simulink model "draft7"  (R2023a)
settings: Solver=VariableStepAuto  StartTime=0.0  StopTime=10  FixedStep=0.0001  MaxStep=0.1  RelTol=1e-3  AbsTol=1e-3  EnableMultiTasking=on
model workspace (MAT data in the model file):
  C_Gimbal = 0.1
  C_IAP = 0.01
  IAP_Pa = 0
  K_Gimbal = 0
  K_IAP = 10
  LeftAbdominalMuscleForce = 0
  LeftBackMuscleForce = 0
  LeftTransverse1MuscleForce = 0
  LeftTransverse2MuscleForce = 0
  Moment_AR = 0
  Moment_FE = 0
  Moment_LB = 0
  RightAbdominalMuscleForce = 0
  RightBackMuscleForce = 0
  RightTransverse1MuscleForce = 0
  RightTransverse2MuscleForce = 0
  a = 1
  b = 1
undefined symbols (not defined in the file): X, Y, Z
libraries: sm_lib x279, nesl_utility x233, simulink_extras x33, checkpacklib x3, simulink x1
(part 2 of 7)

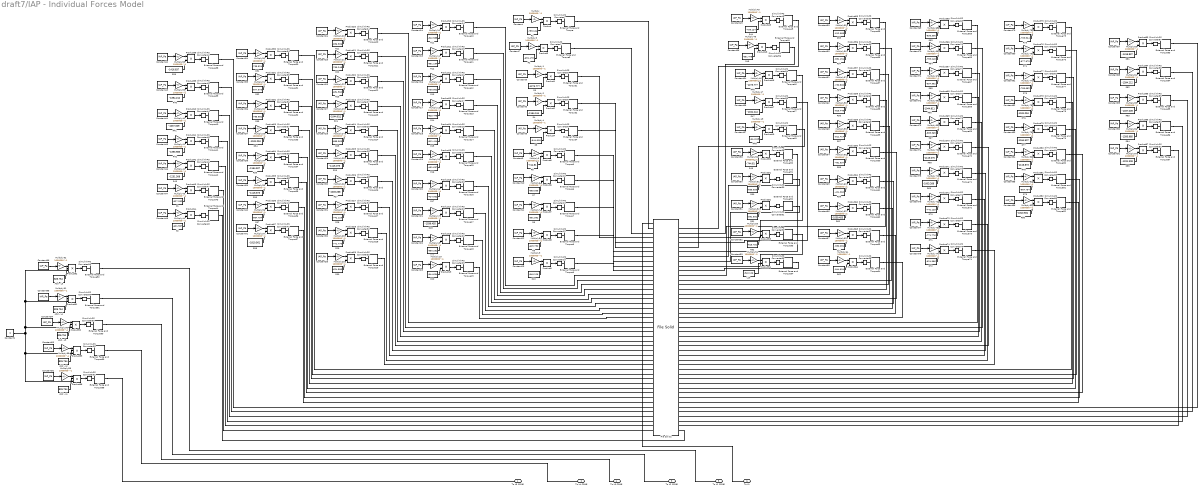
== system draft7/IAP - Individual Forces Model ==
  Abd - L{1..5} (5 alike) : Constant  Value=826.754
  C1 : Constant  Value=-527.332
  C2 : Constant  Value=-621.907
  Constant{,5..96} (93 alike) : Constant  Value=IAP_Pa
  Constant1 : Constant
  External Force and Torque{,1..92} (93 alike) : sm_lib/Forces and Torques/External Force and Torque  ForceResolutionFrame=AttachedFrame  EnableForceX=off  EnableForceY=off  EnableForceZ=on  EnableForce=off  TorqueResolutionFrame=AttachedFrame  EnableTorqueX=off  EnableTorqueY=off  EnableTorqueZ=off  EnableTorque=off
  File Solid2 : sm_lib/Body Elements/File Solid  ExtGeomFileName=C:\Users\siril\OneDrive\Desktop\TIM-Control\Matlab\Simscape models\CAD - with COM\SymmetricModel\draft7\Abd-diamond-flat-solid.step  UnitType=FromFile  ExtGeomFileUnits=m  StepReaderType=HEX  ExportConvexHullGeometry=off  InertiaType=CalculateFromGeometry  Mass=1  MassUnits=kg  CenterOfMass=[0 0 0]  CenterOfMassUnits=m  MomentsOfInertia=[1 1 1]  MomentsOfInertiaUnits=kg*m^2  ProductsOfInertia=[0 0 0]  ProductsOfInertiaUnits=kg*m^2  BasedOnType=Density  Density=0.182  DensityUnits=g/cm^3  DoExposeReferenceFrame=on  SerializedFrames=<Frames><Frame><Id>Frame1</Id><Value><Name>To L1</Name><Origin><Source>GeometricFeature</Source><FeatureName>planar surface 723</FeatureName></Origin><PrimaryAxis><DefinedDirection>-Z</DefinedDirection><Source>GeometricFeature</Source><SourceDirection>+Z</SourceDirection><FeatureName>planar surface 723</FeatureName></PrimaryAxis><SecondaryAxis><DefinedDirection>+X</DefinedDirection><Source>ReferenceFrame</Source><SourceDirection>+X</SourceDirection><FeatureName></FeatureName></SecondaryAxis></Value></Frame><Frame><Id>Frame2</Id><Value><Name>L1</Name><Origin><Source>GeometricFeature</Source><FeatureName>planar surface 1442</FeatureName></Origin><PrimaryAxis><DefinedDirection>+Z</DefinedDirection><Source>GeometricFeature</Source><SourceDirection>+Z</SourceDirection><FeatureName>planar surface 1442</FeatureName></PrimaryAxis><SecondaryAxis><DefinedDirection>+X</DefinedDirection><Source>ReferenceFrame</Source><SourceDirection>+X</SourceDirection><FeatureName></FeatureName></SecondaryAxis></Value></Frame><Frame><Id>Frame3</Id><Value><Name>R1</Name><Origin><Source>GeometricFeature</Source><FeatureName>planar surface 707</FeatureName></Origin><PrimaryAxis><DefinedDirection>-Z</DefinedDirection><Source>GeometricFeature</Source><SourceDirection>+Z</SourceDirection><FeatureName>planar surface 707</FeatureName></PrimaryAxis><SecondaryAxis><DefinedDirection>+X</DefinedDirection><Source>ReferenceFrame</Source><SourceDirection>+X</SourceDirection><FeatureName></FeatureName></SecondaryAxis></Value></Frame><Frame><Id>Frame4</Id><Value><Name>L2</Name><Origin><Source>GeometricFeature</Source><FeatureName>planar surface 1450</FeatureName></Origin><PrimaryAxis><DefinedDirection>+Z</DefinedDirection><Source>GeometricFeature</Source><SourceDirection>+Z</SourceDirection><FeatureName>planar surface 1450</FeatureName></PrimaryAxis><SecondaryAxis><DefinedDirection>+X</DefinedDirection><Source>ReferenceFrame</Source><SourceDirection>+X</SourceDirection><FeatureName></FeatureName></SecondaryAxis></Value></Frame><Frame><Id>Frame5</Id><Value><Name>R2</Name><Origin><Source>GeometricFeature</Source><FeatureName>planar surface 715</FeatureName></Origin><PrimaryAxis><DefinedDirection>-Z</DefinedDirection><Source>GeometricFeature</Source><SourceDirection>+Z</SourceDirection><FeatureName>planar surface 715</FeatureName></PrimaryAxis><SecondaryAxis><DefinedDirection>+X</DefinedDirection><Source>ReferenceFrame</Source><SourceDirection>+X</SourceDirection><FeatureName></FeatureName></SecondaryAxis></Value></Frame><Frame><Id>Frame6</Id><Value><Name>L3</Name><Origin><Source>GeometricFeature</Source><FeatureName>planar surface 1412</FeatureName></Origin><PrimaryAxis><DefinedDirection>+Z</DefinedDirection><Source>GeometricFeature</Source><SourceDirection>+Z</SourceDirection><FeatureName>planar surface 1412</FeatureName></PrimaryAxis><SecondaryAxis><DefinedDirection>+X</DefinedDirection><Source>ReferenceFrame</Source><SourceDirection>+X</SourceDirection><FeatureName></FeatureName></SecondaryAxis></Value></Frame><Frame><Id>Frame7</Id><Value><Name>R3</Name><Origin><Source>GeometricFeature</Source><FeatureName>planar surface 677</FeatureName></Origin><PrimaryAxis><DefinedDirection>-Z</DefinedDirection><Source>GeometricFeature</Source><SourceDirection>+Z</SourceDirection><FeatureName>planar surface 677</FeatureName></PrimaryAxis><SecondaryAxis><DefinedDirection>+X</DefinedDirection><Source>ReferenceFrame</Source><SourceDirection>+X</SourceDirection><FeatureName></FeatureName></SecondaryAxis></Value></Frame><Frame><Id>Frame8</Id><Value><Name>L4</Name><Origin><Source>GeometricFeature</Source><FeatureName>planar surface 1159</FeatureName></Origin><PrimaryAxis><DefinedDirection>+Z</DefinedDirection><Source>GeometricFeature</Source><SourceDirection>+Z</SourceDirection><FeatureName>planar surface 1159</FeatureName></PrimaryAxis><SecondaryAxis><DefinedDirection>+X</DefinedDirection><Source>ReferenceFrame</Source><SourceDirection>+X</SourceDirection><FeatureName></FeatureName></SecondaryAxis></Value></Frame><Frame><Id>Frame9</Id><Value><Name>R4</Name><Origin><Source>GeometricFeature</Source><FeatureName>planar surface 431</FeatureName></Origin><PrimaryAxis><DefinedDirection>-Z</DefinedDirection><Source>GeometricFeature</Source><SourceDirection>+Z</SourceDirection><FeatureName>planar surface 431</FeatureName></PrimaryAxis><SecondaryAxis><DefinedDirection>+X</DefinedDirection><Source>ReferenceFrame</Source><SourceDirection>+X</SourceDirection><FeatureName></FeatureName></SecondaryAxis></Value></Frame><Frame><Id>Frame10</Id><Value><Name>L5</Name><Origin><Source>GeometricFeature</Source><FeatureName>planar surface 1433</FeatureName></Origin><PrimaryAxis><DefinedDirection>+Z</DefinedDirection><Source>GeometricFeature</Source><SourceDirection>+Z</SourceDirection><FeatureName>planar surface 1433</FeatureName></PrimaryAxis><SecondaryAxis><DefinedDirection>+X</DefinedDirection><Source>ReferenceFrame</Source><SourceDirection>+X</SourceDirection><FeatureName></FeatureName></SecondaryAxis></Value></Frame><Frame><Id>Frame11</Id><Value><Name>R5</Name><Origin><Source>GeometricFeature</Source><FeatureName>planar surface 698</FeatureName></Origin><PrimaryAxis><DefinedDirection>-Z</DefinedDirection><Source>GeometricFeature</Source><SourceDirection>+Z</SourceDirection><FeatureName>planar surface 698</FeatureName></PrimaryAxis><SecondaryAxis><DefinedDirection>+X</DefinedDirection><Source>ReferenceFrame</Source><SourceDirection>+X</SourceDirection><FeatureName></FeatureName></SecondaryAxis></Value></Frame><Frame><Id>Frame12</Id><Value><Name>L6</Name><Origin><Source>GeometricFeature</Source><FeatureName>planar surface 1135</FeatureName></Origin><PrimaryAxis><DefinedDirection>+Z</DefinedDirection><Source>GeometricFeature</Source><SourceDirection>+Z</SourceDirection><FeatureName>planar surface 1135</FeatureName></PrimaryAxis><SecondaryAxis><DefinedDirection>+X</DefinedDirection><Source>ReferenceFrame</Source><SourceDirection>+X</SourceDirection><FeatureName></FeatureName></SecondaryAxis></Value></Frame><Frame><Id>Frame13</Id><Value><Name>R6</Name><Origin><Source>GeometricFeature</Source><FeatureName>planar surface 407</FeatureName></Origin><PrimaryAxis><DefinedDirection>-Z</DefinedDirection><Source>GeometricFeature</Source><SourceDirection>+Z</SourceDirection><FeatureName>planar surface 407</FeatureName></PrimaryAxis><SecondaryAxis><DefinedDirection>+X</DefinedDirection><Source>ReferenceFrame</Source><SourceDirection>+X</SourceDirection><FeatureName></FeatureName></SecondaryAxis></Value></Frame><Frame><Id>Frame14</Id><Value><Name>L7</Name><Origin><Source>GeometricFeature</Source><FeatureName>planar surface 1217</FeatureName></Origin><PrimaryAxis><DefinedDirection>+Z</DefinedDirection><Source>GeometricFeature</Source><SourceDirection>+Z</SourceDirection><FeatureName>planar surface 1217</FeatureName></PrimaryAxis><SecondaryAxis><DefinedDirection>+X</DefinedDirection><Source>ReferenceFrame</Source><SourceDirection>+X</SourceDirection><FeatureName></FeatureName></SecondaryAxis></Value></Frame><Frame><Id>Frame15</Id><Value><Name>R7</Name><Origin><Source>GeometricFeature</Source><FeatureName>planar surface 482</FeatureName></Origin><PrimaryAxis><DefinedDirection>-Z</DefinedDirection><Source>GeometricFeature</Source><SourceDirection>+Z</SourceDirection><FeatureName>planar surface 482</FeatureName></PrimaryAxis><SecondaryAxis><DefinedDirection>+X</DefinedDirection><Source>ReferenceFrame</Source><SourceDirection>+X</SourceDirection><FeatureName></FeatureName></SecondaryAxis></Value></Frame><Frame><Id>Frame16</Id><Value><Name>L8</Name><Origin><Source>GeometricFeature</Source><FeatureName>planar surface 1125</FeatureName></Origin><PrimaryAxis><DefinedDirection>+Z</DefinedDirection><Source>GeometricFeature</Source><SourceDirection>+Z</SourceDirection><FeatureName>planar surface 1125</FeatureName></PrimaryAxis><SecondaryAxis><DefinedDirection>+X</DefinedDirection><Source>ReferenceFrame</Source><SourceDirection>+X</SourceDirection><FeatureName></FeatureName></SecondaryAxis></Value></Frame><Frame><Id>Frame17</Id><Value><Name>R8</Name><Origin><Source>GeometricFeature</Source><FeatureName>planar surface 397</FeatureName></Origin><PrimaryAxis><DefinedDirection>-Z</DefinedDirection><Source>GeometricFeature</Source><SourceDirection>+Z</SourceDirection><FeatureName>planar surface 397</FeatureName></PrimaryAxis><SecondaryAxis><DefinedDirection>+X</DefinedDirection><Source>ReferenceFrame</Source><SourceDirection>+X</SourceDirection><FeatureName></FeatureName></SecondaryAxis></Value></Frame><Frame><Id>Frame18</Id><Value><Name>L9</Name><Origin><Source>GeometricFeature</Source><FeatureName>planar surface 1123</FeatureName></Origin><PrimaryAxis><DefinedDirection>+Z</DefinedDirection><Source>GeometricFeature</Source><SourceDirection>+Z</SourceDirection><FeatureName>planar surface 1123</FeatureName></PrimaryAxis><SecondaryAxis><DefinedDirection>+X</DefinedDirection><Source>ReferenceFrame</Source><SourceDirection>+X</SourceDirection><FeatureName></FeatureName></SecondaryAxis></Value></Frame><Frame><Id>Frame19</Id><Value><Name>R9</Name><Origin><Source>GeometricFeature</Source><FeatureName>planar surface 395</FeatureName></Origin><PrimaryAxis><DefinedDirection>-Z</DefinedDirection><Source>GeometricFeature</Source><SourceDirection>+Z</SourceDirection><FeatureName>planar surface 395</FeatureName></PrimaryAxis><SecondaryAxis><DefinedDirection>+X</DefinedDirection><Source>ReferenceFrame</Source><SourceDirection>+X</SourceDirection><FeatureName></FeatureName></SecondaryAxis></Value></Frame><Frame><Id>Frame20</Id><Value><Name>L10</Name><Origin><Source>GeometricFeature</Source><FeatureName>planar surface 1120</FeatureName></Origin><PrimaryAxis><DefinedDirection>+Z</DefinedDirection><Source>GeometricFeature</Source><SourceDirection>+Z</SourceDirection><FeatureName>planar surface 1120</FeatureName></PrimaryAxis><SecondaryAxis><DefinedDirection>+X</DefinedDirection><Source>ReferenceFrame</Source><SourceDirection>+X</SourceDirection><FeatureName></FeatureName></SecondaryAxis></Value></Frame><Frame><Id>Frame21</Id><Value><Name>R10</Name><Origin><Source>GeometricFeature</Source><FeatureName>planar surface 392</FeatureName></Origin><PrimaryAxis><DefinedDirection>-Z</DefinedDirection><Source>GeometricFeature</Source><SourceDirection>+Z</SourceDirection><FeatureName>planar surface 392</FeatureName></PrimaryAxis><SecondaryAxis><DefinedDirection>+X</DefinedDirection><Source>ReferenceFrame</Source><SourceDirection>+X</SourceDirection><FeatureName></FeatureName></SecondaryAxis></Value></Frame><Frame><Id>Frame22</Id><Value><Name>L11</Name><Origin><Source>GeometricFeature</Source><FeatureName>planar surface 1182</FeatureName></Origin><PrimaryAxis><DefinedDirection>+Z</DefinedDirection><Source>GeometricFeature</Source><SourceDirection>+Z</SourceDirection><FeatureName>planar surface 1182</FeatureName></PrimaryAxis><SecondaryAxis><DefinedDirection>+X</DefinedDirection><Source>ReferenceFrame</Source><SourceDirection>+X</SourceDirection><FeatureName></FeatureName></SecondaryAxis></Value></Frame><Frame><Id>Frame23</Id><Value><Name>R11</Name><Origin><Source>GeometricFeature</Source><FeatureName>planar surface 452</FeatureName></Origin><PrimaryAxis><DefinedDirection>-Z</DefinedDirection><Source>GeometricFeature</Source><SourceDirection>+Z</SourceDirection><FeatureName>planar surface 452</FeatureName></PrimaryAxis><SecondaryAxis><DefinedDirection>+X</DefinedDirection><Source>ReferenceFrame</Source><SourceDirection>+X</SourceDirection><FeatureName></FeatureName></SecondaryAxis></Value></Frame><Frame><Id>Frame24</Id><Value><Name>L12</Name><Origin><Source>GeometricFeature</Source><FeatureName>planar surface 1305</FeatureName></Origin><PrimaryAxis><DefinedDirection>+Z</DefinedDirection><Source>GeometricFeature</Source><SourceDirection>+Z</SourceDirection><FeatureName>planar surface 1305</FeatureName></PrimaryAxis><SecondaryAxis><DefinedDirection>+X</DefinedDirection><Source>ReferenceFrame</Source><SourceDirection>+X</SourceDirection><FeatureName></FeatureName></SecondaryAxis></Value></Frame><Frame><Id>Frame25</Id><Value><Name>R12</Name><Origin><Source>GeometricFeature</Source><FeatureName>planar surface 570</FeatureName></Origin><PrimaryAxis><DefinedDirection>-Z</DefinedDirection><Source>GeometricFeature</Source><SourceDirection>+Z</SourceDirection><FeatureName>planar surface 570</FeatureName></PrimaryAxis><SecondaryAxis><DefinedDirection>+X</DefinedDirection><Source>ReferenceFrame</Source><SourceDirection>+X</SourceDirection><FeatureName></FeatureName></SecondaryAxis></Value></Frame><Frame><Id>Frame26</Id><Value><Name>L13</Name><Origin><Source>GeometricFeature</Source><FeatureName>planar surface 1216</FeatureName></Origin><PrimaryAxis><DefinedDirection>+Z</DefinedDirection><Source>GeometricFeature</Source><SourceDirection>+Z</SourceDirection><FeatureName>planar surface 1216</FeatureName></PrimaryAxis><SecondaryAxis><DefinedDirection>+X</DefinedDirection><Source>ReferenceFrame</Source><SourceDirection>+X</SourceDirection><FeatureName></FeatureName></SecondaryAxis></Value></Frame><Frame><Id>Frame27</Id><Value><Name>R13</Name><Origin><Source>GeometricFeature</Source><FeatureName>planar surface 481</FeatureName></Origin><PrimaryAxis><DefinedDirection>-Z</DefinedDirection><Source>GeometricFeature</Source><SourceDirection>+Z</SourceDirection><FeatureName>planar surface 481</FeatureName></PrimaryAxis><SecondaryAxis><DefinedDirection>+X</DefinedDirection><Source>ReferenceFrame</Source><SourceDirection>+X</SourceDirection><FeatureName></FeatureName></SecondaryAxis></Value></Frame><Frame><Id>Frame28</Id><Value><Name>L14</Name><Origin><Source>GeometricFeature</Source><FeatureName>planar surface 1062</FeatureName></Origin><PrimaryAxis><DefinedDirection>+Z</DefinedDirection><Source>GeometricFeature</Source><SourceDirection>+Z</SourceDirection><FeatureName>planar surface 1062</FeatureName></PrimaryAxis><SecondaryAxis><DefinedDirection>+X</DefinedDirection><Source>ReferenceFrame</Source><SourceDirection>+X</SourceDirection><FeatureName></FeatureName></SecondaryAxis></Value></Frame><Frame><Id>Frame29</Id><Value><Name>R14</Name><Origin><Source>GeometricFeature</Source><FeatureName>planar surface 334</FeatureName></Origin><PrimaryAxis><DefinedDirection>-Z</DefinedDirection><Source>GeometricFeature</Source><SourceDirection>+Z</SourceDirection><FeatureName>planar surface 334</FeatureName></PrimaryAxis><SecondaryAxis><DefinedDirection>+X</DefinedDirection><Source>ReferenceFrame</Source><SourceDirection>+X</SourceDirection><FeatureName></FeatureName></SecondaryAxis></Value></Frame><Frame><Id>Frame30</Id><Value><Name>L15</Name><Origin><Source>GeometricFeature</Source><FeatureName>planar surface 1242</FeatureName></Origin><PrimaryAxis><DefinedDirection>+Z</DefinedDirection><Source>GeometricFeature</Source><SourceDirection>+Z</SourceDirection><FeatureName>planar surface 1242</FeatureName></PrimaryAxis><SecondaryAxis><DefinedDirection>+X</DefinedDirection><Source>ReferenceFrame</Source><SourceDirection>+X</SourceDirection><FeatureName></FeatureName></SecondaryAxis></Value></Frame><Frame><Id>Frame31</Id><Value><Name>R15</Name><Origin><Source>GeometricFeature</Source><FeatureName>planar surface 507</FeatureName></Origin><PrimaryAxis><DefinedDirection>-Z</DefinedDirection><Source>GeometricFeature</Source><SourceDirection>+Z</SourceDirection><FeatureName>planar surface 507</FeatureName></PrimaryAxis><SecondaryAxis><DefinedDirection>+X</DefinedDirection><Source>ReferenceFrame</Source><SourceDirection>+X</SourceDirection><FeatureName></FeatureName></SecondaryAxis></Value></Frame><Frame><Id>Frame32</Id><Value><Name>L16</Name><Origin><Source>GeometricFeature</Source><FeatureName>planar surface 1026</FeatureName></Origin><PrimaryAxis><DefinedDirection>+Z</DefinedDirection><Source>GeometricFeature</Source><SourceDirection>+Z</SourceDirection><FeatureName>planar surface 1026</FeatureName></PrimaryAxis><SecondaryAxis><DefinedDirection>+X</DefinedDirection><Source>ReferenceFrame</Source><SourceDirection>+X</SourceDirection><FeatureName></FeatureName></SecondaryAxis></Value></Frame><Frame><Id>Frame33</Id><Value><Name>R16</Name><Origin><Source>GeometricFeature</Source><FeatureName>planar surface 298</FeatureName></Origin><PrimaryAxis><DefinedDirection>-Z</DefinedDirection><Source>GeometricFeature</Source><SourceDirection>+Z</SourceDirection><FeatureName>planar surface 298</FeatureName></PrimaryAxis><SecondaryAxis><DefinedDirection>+X</DefinedDirection><Source>ReferenceFrame</Source><SourceDirection>+X</SourceDirection><FeatureName></FeatureName></SecondaryAxis></Value></Frame><Frame><Id>Frame34</Id><Value><Name>L17</Name><Origin><Source>GeometricFeature</Source><FeatureName>planar surface 1339</FeatureName></Origin><PrimaryAxis><DefinedDirection>+Z</DefinedDirection><Source>GeometricFeature</Source><SourceDirection>+Z</SourceDirection><FeatureName>planar surface 1339</FeatureName></PrimaryAxis><SecondaryAxis><DefinedDirection>+X</DefinedDirection><Source>ReferenceFrame</Source><SourceDirection>+X</SourceDirection><FeatureName></FeatureName></SecondaryAxis></Value></Frame><Frame><Id>Frame35</Id><Value><Name>R17</Name><Origin><Source>GeometricFeature</Source><FeatureName>planar surface 604</FeatureName></Origin><PrimaryAxis><DefinedDirection>-Z</DefinedDirection><Source>GeometricFeature</Source><SourceDirection>+Z</SourceDirection><FeatureName>planar surface 604</FeatureName></PrimaryAxis><SecondaryAxis><DefinedDirection>+X</DefinedDirection><Source>ReferenceFrame</Source><SourceDirection>+X</SourceDirection><FeatureName></FeatureName></SecondaryAxis></Value></Frame><Frame><Id>Frame36</Id><Value><Name>L18</Name><Origin><Source>GeometricFeature</Source><FeatureName>planar surface 1004</FeatureName></Origin><PrimaryAxis><DefinedDirection>+Z</DefinedDirection><Source>GeometricFeature</Source><SourceDirection>+Z</SourceDirection><FeatureName>planar surface 1004</FeatureName></PrimaryAxis><SecondaryAxis><DefinedDirection>+X</DefinedDirection><Source>ReferenceFrame</Source><SourceDirection>+X</SourceDirection><FeatureName></FeatureName></SecondaryAxis></Value></Frame><Frame><Id>Frame37</Id><Value><Name>R18</Name><Origin><Source>GeometricFeature</Source><FeatureName>planar surface 276</FeatureName></Origin><PrimaryAxis><DefinedDirection>-Z</DefinedDirection><Source>GeometricFeature</Source><SourceDirection>+Z</SourceDirection><FeatureName>planar surface 276</FeatureName></PrimaryAxis><SecondaryAxis><DefinedDirection>+X</DefinedDirection><Source>ReferenceFrame</Source><SourceDirection>+X</SourceDirection><FeatureName></FeatureName></SecondaryAxis></Value></Frame><Frame><Id>Frame38</Id><Value><Name>L19</Name><Origin><Source>GeometricFeature</Source><FeatureName>planar surface 996</FeatureName></Origin><PrimaryAxis><DefinedDirection>+Z</DefinedDirection><Source>GeometricFeature</Source><SourceDirection>+Z</SourceDirection><FeatureName>planar surface 996</FeatureName></PrimaryAxis><SecondaryAxis><DefinedDirection>+X</DefinedDirection><Source>ReferenceFrame</Source><SourceDirection>+X</SourceDirection><FeatureName></FeatureName></SecondaryAxis></Value></Frame><Frame><Id>Frame39</Id><Value><Name>R19</Name><Origin><Source>GeometricFeature</Source><FeatureName>planar surface 268</FeatureName></Origin><PrimaryAxis><DefinedDirection>-Z</DefinedDirection><Source>GeometricFeature</Source><SourceDirection>+Z</SourceDirection><FeatureName>planar surface 268</FeatureName></PrimaryAxis><SecondaryAxis><DefinedDirection>+X</DefinedDirection><Source>ReferenceFrame</Source><SourceDirection>+X</SourceDirection><FeatureName></FeatureName></SecondaryAxis></Value></Frame><Frame><Id>Frame40</Id><Value><Name>L20</Name><Origin><Source>GeometricFeature</Source><FeatureName>planar surface 987</FeatureName></Origin><PrimaryAxis><DefinedDirection>+Z</DefinedDirection><Source>GeometricFeature</Source><SourceDirection>+Z</SourceDirection><FeatureName>planar surface 987</FeatureName></PrimaryAxis><SecondaryAxis><DefinedDirection>+X</DefinedDirection><Source>ReferenceFrame</Source><SourceDirection>+X</SourceDirection><FeatureName></FeatureName></SecondaryAxis></Value></Frame><Frame><Id>Frame41</Id><Value><Name>R20</Name><Origin><Source>GeometricFeature</Source><FeatureName>planar surface 259</FeatureName></Origin><PrimaryAxis><DefinedDirection>-Z</DefinedDirection><Source>GeometricFeature</Source><SourceDirection>+Z</SourceDirection><FeatureName>planar surface 259</FeatureName></PrimaryAxis><SecondaryAxis><DefinedDirection>+X</DefinedDirection><Source>ReferenceFrame</Source><SourceDirection>+X</SourceDirection><FeatureName></FeatureName></SecondaryAxis></Value></Frame><Frame><Id>Frame42</Id><Value><Name>L21</Name><Origin><Source>GeometricFeature</Source><FeatureName>planar surface 1218</FeatureName></Origin><PrimaryAxis><DefinedDirection>+Z</DefinedDirection><Source>GeometricFeature</Source><SourceDirection>+Z</SourceDirection><FeatureName>planar surface 1218</FeatureName></PrimaryAxis><SecondaryAxis><DefinedDirection>+X</DefinedDirection><Source>ReferenceFrame</Source><SourceDirection>+X</SourceDirection><FeatureName></FeatureName></SecondaryAxis></Value></Frame><Frame><Id>Frame43</Id><Value><Name>R21</Name><Origin><Source>GeometricFeature</Source><FeatureName>planar surface 483</FeatureName></Origin><PrimaryAxis><DefinedDirection>-Z</DefinedDirection><Source>GeometricFeature</Source><SourceDirection>+Z</SourceDirection><FeatureName>planar surface 483</FeatureName></PrimaryAxis><SecondaryAxis><DefinedDirection>+X</DefinedDirection><Source>ReferenceFrame</Source><SourceDirection>+X</SourceDirection><FeatureName></FeatureName></SecondaryAxis></Value></Frame><Frame><Id>Frame44</Id><Value><Name>L22</Name><Origin><Source>GeometricFeature</Source><FeatureName>planar surface 1364</FeatureName></Origin><PrimaryAxis><DefinedDirection>+Z</DefinedDirection><Source>GeometricFeature</Source><SourceDirection>+Z</SourceDirection><FeatureName>planar surface 1364</FeatureName></PrimaryAxis><SecondaryAxis><DefinedDirection>+X</DefinedDirection><Source>ReferenceFrame</Source><SourceDirection>+X</SourceDirection><FeatureName></FeatureName></SecondaryAxis></Value></Frame><Frame><Id>Frame45</Id><Value><Name>R22</Name><Origin><Source>GeometricFeature</Source><FeatureName>planar surface 629</FeatureName></Origin><PrimaryAxis><DefinedDirection>-Z</DefinedDirection><Source>GeometricFeature</Source><SourceDirection>+Z</SourceDirection><FeatureName>planar surface 629</FeatureName></PrimaryAxis><SecondaryAxis><DefinedDirection>+X</DefinedDirection><Source>ReferenceFrame</Source><SourceDirection>+X</SourceDirection><FeatureName></FeatureName></SecondaryAxis></Value></Frame><Frame><Id>Frame46</Id><Value><Name>L23</Name><Origin><Source>GeometricFeature</Source><FeatureName>planar surface 1381</FeatureName></Origin><PrimaryAxis><DefinedDirection>+Z</DefinedDirection><Source>GeometricFeature</Source><SourceDirection>+Z</SourceDirection><FeatureName>planar surface 1381</FeatureName></PrimaryAxis><SecondaryAxis><DefinedDirection>+X</DefinedDirection><Source>ReferenceFrame</Source><SourceDirection>+X</SourceDirection><FeatureName></FeatureName></SecondaryAxis></Value></Frame><Frame><Id>Frame47</Id><Value><Name>R23</Name><Origin><Source>GeometricFeature</Source><FeatureName>planar surface 646</FeatureName></Origin><PrimaryAxis><DefinedDirection>-Z</DefinedDirection><Source>GeometricFeature</Source><SourceDirection>+Z</SourceDirection><FeatureName>planar surface 646</FeatureName></PrimaryAxis><SecondaryAxis><DefinedDirection>+X</DefinedDirection><Source>ReferenceFrame</Source><SourceDirection>+X</SourceDirection><FeatureName></FeatureName></SecondaryAxis></Value></Frame><Frame><Id>Frame48</Id><Value><Name>L24</Name><Origin><Source>GeometricFeature</Source><FeatureName>planar surface 950</FeatureName></Origin><PrimaryAxis><DefinedDirection>+Z</DefinedDirection><Source>GeometricFeature</Source><SourceDirection>+Z</SourceDirection><FeatureName>planar surface 950</FeatureName></PrimaryAxis><SecondaryAxis><DefinedDirection>+X</DefinedDirection><Source>ReferenceFrame</Source><SourceDirection>+X</SourceDirection><FeatureName></FeatureName></SecondaryAxis></Value></Frame><Frame><Id>Frame49</Id><Value><Name>R24</Name><Origin><Source>GeometricFeature</Source><FeatureName>planar surface 222</FeatureName></Origin><PrimaryAxis><DefinedDirection>-Z</DefinedDirection><Source>GeometricFeature</Source><SourceDirection>+Z</SourceDirection><FeatureName>planar surface 222</FeatureName></PrimaryAxis><SecondaryAxis><DefinedDirection>+X</DefinedDirection><Source>ReferenceFrame</Source><SourceDirection>+X</SourceDirection><FeatureName></FeatureName></SecondaryAxis></Value></Frame><Frame><Id>Frame50</Id><Value><Name>L25</Name><Origin><Source>GeometricFeature</Source><FeatureName>planar surface 1231</FeatureName></Origin><PrimaryAxis><DefinedDirection>+Z</DefinedDirection><Source>GeometricFeature</Source><SourceDirection>+Z</SourceDirection><FeatureName>planar surface 1231</FeatureName></PrimaryAxis><SecondaryAxis><DefinedDirection>+X</DefinedDirection><Source>ReferenceFrame</Source><SourceDirection>+X</SourceDirection><FeatureName></FeatureName></SecondaryAxis></Value></Frame><Frame><Id>Frame51</Id><Value><Name>R25</Name><Origin><Source>GeometricFeature</Source><FeatureName>planar surface 496</FeatureName></Origin><PrimaryAxis><DefinedDirection>-Z</DefinedDirection><Source>GeometricFeature</Source><SourceDirection>+Z</SourceDirection><FeatureName>planar surface 496</FeatureName></PrimaryAxis><SecondaryAxis><DefinedDirection>+X</DefinedDirection><Source>ReferenceFrame</Source><SourceDirection>+X</SourceDirection><FeatureName></FeatureName></SecondaryAxis></Value></Frame><Frame><Id>Frame52</Id><Value><Name>L26</Name><Origin><Source>GeometricFeature</Source><FeatureName>planar surface 916</FeatureName></Origin><PrimaryAxis><DefinedDirection>+Z</DefinedDirection><Source>GeometricFeature</Source><SourceDirection>+Z</SourceDirection><FeatureName>planar surface 916</FeatureName></PrimaryAxis><SecondaryAxis><DefinedDirection>+X</DefinedDirection><Source>ReferenceFrame</Source><SourceDirection>+X</SourceDirection><FeatureName></FeatureName></SecondaryAxis></Value></Frame><Frame><Id>Frame53</Id><Value><Name>R26</Name><Origin><Source>GeometricFeature</Source><FeatureName>planar surface 188</FeatureName></Origin><PrimaryAxis><DefinedDirection>-Z</DefinedDirection><Source>GeometricFeature</Source><SourceDirection>+Z</SourceDirection><FeatureName>planar surface 188</FeatureName></PrimaryAxis><SecondaryAxis><DefinedDirection>+X</DefinedDirection><Source>ReferenceFrame</Source><SourceDirection>+X</SourceDirection><FeatureName></FeatureName></SecondaryAxis></Value></Frame><Frame><Id>Frame54</Id><Value><Name>L27</Name><Origin><Source>GeometricFeature</Source><FeatureName>planar surface 1358</FeatureName></Origin><PrimaryAxis><DefinedDirection>+Z</DefinedDirection><Source>GeometricFeature</Source><SourceDirection>+Z</SourceDirection><FeatureName>planar surface 1358</FeatureName></PrimaryAxis><SecondaryAxis><DefinedDirection>+X</DefinedDirection><Source>ReferenceFrame</Source><SourceDirection>+X</SourceDirection><FeatureName></FeatureName></SecondaryAxis></Value></Frame><Frame><Id>Frame55</Id><Value><Name>R27</Name><Origin><Source>GeometricFeature</Source><FeatureName>planar surface 623</FeatureName></Origin><PrimaryAxis><DefinedDirection>-Z</DefinedDirection><Source>GeometricFeature</Source><SourceDirection>+Z</SourceDirection><FeatureName>planar surface 623</FeatureName></PrimaryAxis><SecondaryAxis><DefinedDirection>+X</DefinedDirection><Source>ReferenceFrame</Source><SourceDirection>+X</SourceDirection><FeatureName></FeatureName></SecondaryAxis></Value></Frame><Frame><Id>Frame56</Id><Value><Name>L28</Name><Origin><Source>GeometricFeature</Source><FeatureName>planar surface 896</FeatureName></Origin><PrimaryAxis><DefinedDirection>+Z</DefinedDirection><Source>GeometricFeature</Source><SourceDirection>+Z</SourceDirection><FeatureName>planar surface 896</FeatureName></PrimaryAxis><SecondaryAxis><DefinedDirection>+X</DefinedDirection><Source>ReferenceFrame</Source><SourceDirection>+X</SourceDirection><FeatureName></FeatureName></SecondaryAxis></Value></Frame><Frame><Id>Frame57</Id><Value><Name>R28</Name><Origin><Source>GeometricFeature</Source><FeatureName>planar surface 168</FeatureName></Origin><PrimaryAxis><DefinedDirection>-Z</DefinedDirection><Source>GeometricFeature</Source><SourceDirection>+Z</SourceDirection><FeatureName>planar surface 168</FeatureName></PrimaryAxis><SecondaryAxis><DefinedDirection>+X</DefinedDirection><Source>ReferenceFrame</Source><SourceDirection>+X</SourceDirection><FeatureName></FeatureName></SecondaryAxis></Value></Frame><Frame><Id>Frame58</Id><Value><Name>L29</Name><Origin><Source>GeometricFeature</Source><FeatureName>planar surface 889</FeatureName></Origin><PrimaryAxis><DefinedDirection>+Z</DefinedDirection><Source>GeometricFeature</Source><SourceDirection>+Z</SourceDirection><FeatureName>planar surface 889</FeatureName></PrimaryAxis><SecondaryAxis><DefinedDirection>+X</DefinedDirection><Source>ReferenceFrame</Source><SourceDirection>+X</SourceDirection><FeatureName></FeatureName></SecondaryAxis></Value></Frame><Frame><Id>Frame59</Id><Value><Name>R29</Name><Origin><Source>GeometricFeature</Source><FeatureName>planar surface 161</FeatureName></Origin><PrimaryAxis><DefinedDirection>-Z</DefinedDirection><Source>GeometricFeature</Source><SourceDirection>+Z</SourceDirection><FeatureName>planar surface 161</FeatureName></PrimaryAxis><SecondaryAxis><DefinedDirection>+X</DefinedDirection><Source>ReferenceFrame</Source><SourceDirection>+X</SourceDirection><FeatureName></FeatureName></SecondaryAxis></Value></Frame><Frame><Id>Frame60</Id><Value><Name>L30</Name><Origin><Source>GeometricFeature</Source><FeatureName>planar surface 881</FeatureName></Origin><PrimaryAxis><DefinedDirection>+Z</DefinedDirection><Source>GeometricFeature</Source><SourceDirection>+Z</SourceDirection><FeatureName>planar surface 881</FeatureName></PrimaryAxis><SecondaryAxis><DefinedDirection>+X</DefinedDirection><Source>ReferenceFrame</Source><SourceDirection>+X</SourceDirection><FeatureName></FeatureName></SecondaryAxis></Value></Frame><Frame><Id>Frame61</Id><Value><Name>R30</Name><Origin><Source>GeometricFeature</Source><FeatureName>planar surface 153</FeatureName></Origin><PrimaryAxis><DefinedDirection>-Z</DefinedDirection><Source>GeometricFeature</Source><SourceDirection>+Z</SourceDirection><FeatureName>planar surface 153</FeatureName></PrimaryAxis><SecondaryAxis><DefinedDirection>+X</DefinedDirection><Source>ReferenceFrame</Source><SourceDirection>+X</SourceDirection><FeatureName></FeatureName></SecondaryAxis></Value></Frame><Frame><Id>Frame62</Id><Value><Name>L31</Name><Origin><Source>GeometricFeature</Source><FeatureName>planar surface 1280</FeatureName></Origin><PrimaryAxis><DefinedDirection>+Z</DefinedDirection><Source>GeometricFeature</Source><SourceDirection>+Z</SourceDirection><FeatureName>planar surface 1280</FeatureName></PrimaryAxis><SecondaryAxis><DefinedDirection>+X</DefinedDirection><Source>ReferenceFrame</Source><SourceDirection>+X</SourceDirection><FeatureName></FeatureName></SecondaryAxis></Value></Frame><Frame><Id>Frame63</Id><Value><Name>R31</Name><Origin><Source>GeometricFeature</Source><FeatureName>planar surface 545</FeatureName></Origin><PrimaryAxis><DefinedDirection>-Z</DefinedDirection><Source>GeometricFeature</Source><SourceDirection>+Z</SourceDirection><FeatureName>planar surface 545</FeatureName></PrimaryAxis><SecondaryAxis><DefinedDirection>+X</DefinedDirection><Source>ReferenceFrame</Source><SourceDirection>+X</SourceDirection><FeatureName></FeatureName></SecondaryAxis></Value></Frame><Frame><Id>Frame64</Id><Value><Name>L32</Name><Origin><Source>GeometricFeature</Source><FeatureName>planar surface 1224</FeatureName></Origin><PrimaryAxis><DefinedDirection>+Z</DefinedDirection><Source>GeometricFeature</Source><SourceDirection>+Z</SourceDirection><FeatureName>planar surface 1224</FeatureName></PrimaryAxis><SecondaryAxis><DefinedDirection>+X</DefinedDirection><Source>ReferenceFrame</Source><SourceDirection>+X</SourceDirection><FeatureName></FeatureName></SecondaryAxis></Value></Frame><Frame><Id>Frame65</Id><Value><Name>R32</Name><Origin><Source>GeometricFeature</Source><FeatureName>planar surface 489</FeatureName></Origin><PrimaryAxis><DefinedDirection>-Z</DefinedDirection><Source>GeometricFeature</Source><SourceDirection>+Z</SourceDirection><FeatureName>planar surface 489</FeatureName></PrimaryAxis><SecondaryAxis><DefinedDirection>+X</DefinedDirection><Source>ReferenceFrame</Source><SourceDirection>+X</SourceDirection><FeatureName></FeatureName></SecondaryAxis></Value></Frame><Frame><Id>Frame66</Id><Value><Name>L33</Name><Origin><Source>GeometricFeature</Source><FeatureName>planar surface 1400</FeatureName></Origin><PrimaryAxis><DefinedDirection>+Z</DefinedDirection><Source>GeometricFeature</Source><SourceDirection>+Z</SourceDirection><FeatureName>planar surface 1400</FeatureName></PrimaryAxis><SecondaryAxis><DefinedDirection>+X</DefinedDirection><Source>ReferenceFrame</Source><SourceDirection>+X</SourceDirection><FeatureName></FeatureName></SecondaryAxis></Value></Frame><Frame><Id>Frame67</Id><Value><Name>R33</Name><Origin><Source>GeometricFeature</Source><FeatureName>planar surface 665</FeatureName></Origin><PrimaryAxis><DefinedDirection>-Z</DefinedDirection><Source>GeometricFeature</Source><SourceDirection>+Z</SourceDirection><FeatureName>planar surface 665</FeatureName></PrimaryAxis><SecondaryAxis><DefinedDirection>+X</DefinedDirection><Source>ReferenceFrame</Source><SourceDirection>+X</SourceDirection><FeatureName></FeatureName></SecondaryAxis></Value></Frame><Frame><Id>Frame68</Id><Value><Name>L34</Name><Origin><Source>GeometricFeature</Source><FeatureName>planar surface 848</FeatureName></Origin><PrimaryAxis><DefinedDirection>+Z</DefinedDirection><Source>GeometricFeature</Source><SourceDirection>+Z</SourceDirection><FeatureName>planar surface 848</FeatureName></PrimaryAxis><SecondaryAxis><DefinedDirection>+X</DefinedDirection><Source>ReferenceFrame</Source><SourceDirection>+X</SourceDirection><FeatureName></FeatureName></SecondaryAxis></Value></Frame><Frame><Id>Frame69</Id><Value><Name>R34</Name><Origin><Source>GeometricFeature</Source><FeatureName>planar surface 120</FeatureName></Origin><PrimaryAxis><DefinedDirection>-Z</DefinedDirection><Source>GeometricFeature</Source><SourceDirection>+Z</SourceDirection><FeatureName>planar surface 120</FeatureName></PrimaryAxis><SecondaryAxis><DefinedDirection>+X</DefinedDirection><Source>ReferenceFrame</Source><SourceDirection>+X</SourceDirection><FeatureName></FeatureName></SecondaryAxis></Value></Frame><Frame><Id>Frame70</Id><Value><Name>L35</Name><Origin><Source>GeometricFeature</Source><FeatureName>planar surface 1385</FeatureName></Origin><PrimaryAxis><DefinedDirection>+Z</DefinedDirection><Source>GeometricFeature</Source><SourceDirection>+Z</SourceDirection><FeatureName>planar surface 1385</FeatureName></PrimaryAxis><SecondaryAxis><DefinedDirection>+X</DefinedDirection><Source>ReferenceFrame</Source><SourceDirection>+X</SourceDirection><FeatureName></FeatureName></SecondaryAxis></Value></Frame><Frame><Id>Frame71</Id><Value><Name>R35</Name><Origin><Source>GeometricFeature</Source><FeatureName>planar surface 650</FeatureName></Origin><PrimaryAxis><DefinedDirection>-Z</DefinedDirection><Source>GeometricFeature</Source><SourceDirection>+Z</SourceDirection><FeatureName>planar surface 650</FeatureName></PrimaryAxis><SecondaryAxis><DefinedDirection>+X</DefinedDirection><Source>ReferenceFrame</Source><SourceDirection>+X</SourceDirection><FeatureName></FeatureName></SecondaryAxis></Value></Frame><Frame><Id>Frame72</Id><Value><Name>L36</Name><Origin><Source>GeometricFeature</Source><FeatureName>planar surface 816</FeatureName></Origin><PrimaryAxis><DefinedDirection>+Z</DefinedDirection><Source>GeometricFeature</Source><SourceDirection>+Z</SourceDirection><FeatureName>planar surface 816</FeatureName></PrimaryAxis><SecondaryAxis><DefinedDirection>+X</DefinedDirection><Source>ReferenceFrame</Source><SourceDirection>+X</SourceDirection><FeatureName></FeatureName></SecondaryAxis></Value></Frame><Frame><Id>Frame73</Id><Value><Name>R36</Name><Origin><Source>GeometricFeature</Source><FeatureName>planar surface 88</FeatureName></Origin><PrimaryAxis><DefinedDirection>-Z</DefinedDirection><Source>GeometricFeature</Source><SourceDirection>+Z</SourceDirection><FeatureName>planar surface 88</FeatureName></PrimaryAxis><SecondaryAxis><DefinedDirection>+X</DefinedDirection><Source>ReferenceFrame</Source><SourceDirection>+X</SourceDirection><FeatureName></FeatureName></SecondaryAxis></Value></Frame><Frame><Id>Frame74</Id><Value><Name>L37</Name><Origin><Source>GeometricFeature</Source><FeatureName>segment 6127</FeatureName></Origin><PrimaryAxis><DefinedDirection>+Z</DefinedDirection><Source>GeometricFeature</Source><SourceDirection>+Z</SourceDirection><FeatureName>segment 6128</FeatureName></PrimaryAxis><SecondaryAxis><DefinedDirection>+X</DefinedDirection><Source>ReferenceFrame</Source><SourceDirection>+X</SourceDirection><FeatureName></FeatureName></SecondaryAxis></Value></Frame><Frame><Id>Frame75</Id><Value><Name>R37</Name><Origin><Source>GeometricFeature</Source><FeatureName>segment 6112</FeatureName></Origin><PrimaryAxis><DefinedDirection>+Z</DefinedDirection><Source>GeometricFeature</Source><SourceDirection>+Z</SourceDirection><FeatureName>segment 6123</FeatureName></PrimaryAxis><SecondaryAxis><DefinedDirection>+X</DefinedDirection><Source>ReferenceFrame</Source><SourceDirection>+X</SourceDirection><FeatureName></FeatureName></SecondaryAxis></Value></Frame><Frame><Id>Frame76</Id><Value><Name>L38</Name><Origin><Source>GeometricFeature</Source><FeatureName>segment 6294</FeatureName></Origin><PrimaryAxis><DefinedDirection>+Z</DefinedDirection><Source>GeometricFeature</Source><SourceDirection>+Z</SourceDirection><FeatureName>segment 6289</FeatureName></PrimaryAxis><SecondaryAxis><DefinedDirection>+Y</DefinedDirection><Source>ReferenceFrame</Source><SourceDirection>+X</SourceDirection><FeatureName></FeatureName></SecondaryAxis></Value></Frame><Frame><Id>Frame77</Id><Value><Name>R38</Name><Origin><Source>GeometricFeature</Source><FeatureName>segment 6267</FeatureName></Origin><PrimaryAxis><DefinedDirection>+Z</DefinedDirection><Source>GeometricFeature</Source><SourceDirection>+Z</SourceDirection><FeatureName>segment 6282</FeatureName></PrimaryAxis><SecondaryAxis><DefinedDirection>-Y</DefinedDirection><Source>ReferenceFrame</Source><SourceDirection>+X</SourceDirection><FeatureName></FeatureName></SecondaryAxis></Value></Frame><Frame><Id>Frame78</Id><Value><Name>L39</Name><Origin><Source>GeometricFeature</Source><FeatureName>segment 6303</FeatureName></Origin><PrimaryAxis><DefinedDirection>+Z</DefinedDirection><Source>GeometricFeature</Source><SourceDirection>+Z</SourceDirection><FeatureName>segment 6469</FeatureName></PrimaryAxis><SecondaryAxis><DefinedDirection>-Y</DefinedDirection><Source>ReferenceFrame</Source><SourceDirection>+X</SourceDirection><FeatureName></FeatureName></SecondaryAxis></Value></Frame><Frame><Id>Frame79</Id><Value><Name>R39</Name><Origin><Source>GeometricFeature</Source><FeatureName>segment 6263</FeatureName></Origin><PrimaryAxis><DefinedDirection>+Z</DefinedDirection><Source>GeometricFeature</Source><SourceDirection>+Z</SourceDirection><FeatureName>segment 6453</FeatureName></PrimaryAxis><SecondaryAxis><DefinedDirection>+Y</DefinedDirection><Source>ReferenceFrame</Source><SourceDirection>+X</SourceDirection><FeatureName></FeatureName></SecondaryAxis></Value></Frame><Frame><Id>Frame80</Id><Value><Name>L40</Name><Origin><Source>GeometricFeature</Source><FeatureName>planar surface 808</FeatureName></Origin><PrimaryAxis><DefinedDirection>+Z</DefinedDirection><Source>GeometricFeature</Source><SourceDirection>+Z</SourceDirection><FeatureName>planar surface 808</FeatureName></PrimaryAxis><SecondaryAxis><DefinedDirection>+X</DefinedDirection><Source>ReferenceFrame</Source><SourceDirection>+X</SourceDirection><FeatureName></FeatureName></SecondaryAxis></Value></Frame><Frame><Id>Frame81</Id><Value><Name>R40</Name><Origin><Source>GeometricFeature</Source><FeatureName>planar surface 80</FeatureName></Origin><PrimaryAxis><DefinedDirection>-Z</DefinedDirection><Source>GeometricFeature</Source><SourceDirection>+Z</SourceDirection><FeatureName>planar surface 80</FeatureName></PrimaryAxis><SecondaryAxis><DefinedDirection>+X</DefinedDirection><Source>ReferenceFrame</Source><SourceDirection>+X</SourceDirection><FeatureName></FeatureName></SecondaryAxis></Value></Frame><Frame><Id>Frame82</Id><Value><Name>L41</Name><Origin><Source>GeometricFeature</Source><FeatureName>planar surface 791</FeatureName></Origin><PrimaryAxis><DefinedDirection>+Z</DefinedDirection><Source>GeometricFeature</Source><SourceDirection>+Z</SourceDirection><FeatureName>planar surface 791</FeatureName></PrimaryAxis><SecondaryAxis><DefinedDirection>+X</DefinedDirection><Source>ReferenceFrame</Source><SourceDirection>+X</SourceDirection><FeatureName></FeatureName></SecondaryAxis></Value></Frame><Frame><Id>Frame83</Id><Value><Name>R41</Name><Origin><Source>GeometricFeature</Source><FeatureName>planar surface 63</FeatureName></Origin><PrimaryAxis><DefinedDirection>-Z</DefinedDirection><Source>GeometricFeature</Source><SourceDirection>+Z</SourceDirection><FeatureName>planar surface 63</FeatureName></PrimaryAxis><SecondaryAxis><DefinedDirection>+X</DefinedDirection><Source>ReferenceFrame</Source><SourceDirection>+X</SourceDirection><FeatureName></FeatureName></SecondaryAxis></Value></Frame><Frame><Id>Frame84</Id><Value><Name>L42</Name><Origin><Source>GeometricFeature</Source><FeatureName>planar surface 769</FeatureName></Origin><PrimaryAxis><DefinedDirection>+Z</DefinedDirection><Source>GeometricFeature</Source><SourceDirection>+Z</SourceDirection><FeatureName>planar surface 769</FeatureName></PrimaryAxis><SecondaryAxis><DefinedDirection>+X</DefinedDirection><Source>ReferenceFrame</Source><SourceDirection>+X</SourceDirection><FeatureName></FeatureName></SecondaryAxis></Value></Frame><Frame><Id>Frame85</Id><Value><Name>R42</Name><Origin><Source>GeometricFeature</Source><FeatureName>planar surface 41</FeatureName></Origin><PrimaryAxis><DefinedDirection>-Z</DefinedDirection><Source>GeometricFeature</Source><SourceDirection>+Z</SourceDirection><FeatureName>planar surface 41</FeatureName></PrimaryAxis><SecondaryAxis><DefinedDirection>+X</DefinedDirection><Source>ReferenceFrame</Source><SourceDirection>+X</SourceDirection><FeatureName></FeatureName></SecondaryAxis></Value></Frame><Frame><Id>Frame86</Id><Value><Name>L43</Name><Origin><Source>GeometricFeature</Source><FeatureName>segment 3140</FeatureName></Origin><PrimaryAxis><DefinedDirection>+Z</DefinedDirection><Source>GeometricFeature</Source><SourceDirection>+Z</SourceDirection><FeatureName>segment 5809</FeatureName></PrimaryAxis><SecondaryAxis><DefinedDirection>+X</DefinedDirection><Source>ReferenceFrame</Source><SourceDirection>+X</SourceDirection><FeatureName></FeatureName></SecondaryAxis></Value></Frame><Frame><Id>Frame87</Id><Value><Name>R43</Name><Origin><Source>GeometricFeature</Source><FeatureName>segment 85</FeatureName></Origin><PrimaryAxis><DefinedDirection>+Z</DefinedDirection><Source>GeometricFeature</Source><SourceDirection>+Z</SourceDirection><FeatureName>segment 2778</FeatureName></PrimaryAxis><SecondaryAxis><DefinedDirection>+X</DefinedDirection><Source>ReferenceFrame</Source><SourceDirection>+X</SourceDirection><FeatureName></FeatureName></SecondaryAxis></Value></Frame><Frame><Id>Frame88</Id><Value><Name>C1</Name><Origin><Source>GeometricFeature</Source><FeatureName>point 9476</FeatureName></Origin><PrimaryAxis><DefinedDirection>+Z</DefinedDirection><Source>GeometricFeature</Source><SourceDirection>+Z</SourceDirection><FeatureName>segment 2410</FeatureName></PrimaryAxis><SecondaryAxis><DefinedDirection>+X</DefinedDirection><Source>ReferenceFrame</Source><SourceDirection>+X</SourceDirection><FeatureName></FeatureName></SecondaryAxis></Value></Frame><Frame><Id>Frame89</Id><Value><Name>C2</Name><Origin><Source>GeometricFeature</Source><FeatureName>planar surface 1191</FeatureName></Origin><PrimaryAxis><DefinedDirection>-Z</DefinedDirection><Source>GeometricFeature</Source><SourceDirection>+Z</SourceDirection><FeatureName>planar surface 1191</FeatureName></PrimaryAxis><SecondaryAxis><DefinedDirection>+X</DefinedDirection><Source>ReferenceFrame</Source><SourceDirection>+X</SourceDirection><FeatureName></FeatureName></SecondaryAxis></Value></Frame></Frames>  GraphicType=FromGeometry  MarkerShape=Sphere  MarkerSize=10  GraphicVisPropType=SimpleVisualProperties  GraphicDiffuseColor=[0.5 0.5 0.5]  GraphicSpecularColor=[0.5 0.5 0.5 1.0]  GraphicAmbientColor=[0.15 0.15 0.15 1.0]  GraphicEmissiveColor=[0.0 0.0 0.0 1.0]  GraphicShininess=75  GraphicOpacity=1.0
  L10 : Constant  Value=-540.126
  Multiply{,1..92} (93 alike) : Gain  Gain=1000000^-1
  Product{,1..87} (88 alike) : Product
  Product{88..92} (5 alike) : Product  Inputs=3
  R1 : Constant  Value=-759.124
  R10 : Constant  Value=-540.126
  R11 : Constant  Value=-512.985
  R12 : Constant  Value=-951.194
  R13 : Constant  Value=-730.802
  R14 : Constant  Value=-825.448
  R15 : Constant  Value=-511.414
  R16 : Constant  Value=-491.637
  R17 : Constant  Value=-424.062
  R18 : Constant  Value=-1039.455
  R19 : Constant  Value=-950.281
  R2 : Constant  Value=-651.478
  R20 : Constant  Value=-944.634
  R21 : Constant  Value=-836.306
  R22 : Constant  Value=-759.248
  R23 : Constant  Value=-654.962
  R24 : Constant  Value=-1044.811
  R25 : Constant  Value=-885.365
  R26 : Constant  Value=-1115.075
  R27 : Constant  Value=-1003.268
  R28 : Constant  Value=-742.129
  R29 : Constant  Value=-771.776
  R3 : Constant  Value=-1273.777
  R30 : Constant  Value=-624.586
  R31 : Constant  Value=-735.524
  R32 : Constant  Value=-877.973
  R33 : Constant  Value=-785.682
  R34 : Constant  Value=-1181.094
  R35 : Constant  Value=-1164.507
  R36 : Constant  Value=-1116.873
  R37 : Constant  Value=-864.754
  R38 : Constant  Value=-1810.561
  R39 : Constant  Value=-1416.837
  R4 : Constant  Value=-1164.244
  R40 : Constant  Value=-1394.212
  R41 : Constant  Value=-1037.009
  R42 : Constant  Value=-1393.985
  R43 : Constant  Value=-1231.308
  R44 : Constant  Value=-759.124
  R45 : Constant  Value=-651.478
  R46 : Constant  Value=-1273.777
  R47 : Constant  Value=-1164.244
  R48 : Constant  Value=-644.618
  R49 : Constant  Value=-744.81
  R5 : Constant  Value=-644.618
  R50 : Constant  Value=-665.935
  R51 : Constant  Value=-391.592
  R52 : Constant  Value=-615.752
  R53 : Constant  Value=-512.985
  R54 : Constant  Value=-951.194
  R55 : Constant  Value=-730.802
  R56 : Constant  Value=-825.448
  R57 : Constant  Value=-511.414
  R58 : Constant  Value=-491.637
  R59 : Constant  Value=-424.062
  R6 : Constant  Value=-744.81
  R60 : Constant  Value=-1039.455
  R61 : Constant  Value=-950.281
  R62 : Constant  Value=-944.634
  R63 : Constant  Value=-836.306
  R64 : Constant  Value=-759.248
  R65 : Constant  Value=-654.962
  R66 : Constant  Value=-1044.811
  R67 : Constant  Value=-885.365
  R68 : Constant  Value=-1115.075
  R69 : Constant  Value=-1003.268
  R7 : Constant  Value=-665.935
  R70 : Constant  Value=-742.129
  R71 : Constant  Value=-771.776
  R72 : Constant  Value=-624.586
  R73 : Constant  Value=-735.524
  R74 : Constant  Value=-877.973
  R75 : Constant  Value=-785.682
  R76 : Constant  Value=-1181.094
  R77 : Constant  Value=-1164.507
  R78 : Constant  Value=-1116.873
  R79 : Constant  Value=-864.754
  R8 : Constant  Value=-391.592
  R80 : Constant  Value=-1810.561
  R81 : Constant  Value=-1416.837
  R82 : Constant  Value=-1394.212
  R83 : Constant  Value=-1037.009
  R84 : Constant  Value=-1393.985
  R85 : Constant  Value=-1231.308
  R9 : Constant  Value=-615.752
  Simulink-PS Converter{,5..96} (93 alike) : nesl_utility/Simulink-PS Converter  PhysicalDomain=network_engine_domain  SubClassName=ps_input  LeftPortType=input  RightPortType=output  PseudoPeriodic=off  Frequencies=[]  NoiseDistribution=none  NoiseParameters=[]  Unit=1  AffineConversion=off  FilteringAndDerivatives=provide  SimscapeFilterOrder=1  InputFilterTimeConstant=0.001  UdotUserProvided=0
  To L5 CONE : PMIOPort  Side=Right
  To L4 CONE : PMIOPort  Port=2  Side=Right
  To L2 CONE : PMIOPort  Port=3  Side=Right
  To L3 CONE : PMIOPort  Port=4  Side=Right
  To L1 CONE : PMIOPort  Port=5  Side=Right
  To L1 : PMIOPort  Port=6  Side=Left
  wires:
  R78/1 -> Product80/2
  Multiply23/1 -> Product23/1
  Constant8/1 -> Multiply4/1
  Multiply45/1 -> Product45/1
  Constant85/1 -> Multiply81/1
  Constant95/1 -> Multiply91/1
  C1/1 -> Product43/2
  Product17/1 -> Simulink-PS Converter21/1
  Multiply14/1 -> Product14/1
  Constant33/1 -> Multiply29/1
  Product34/1 -> Simulink-PS Converter38/1
  Product52/1 -> Simulink-PS Converter51/1
  R67/1 -> Product69/2
  R15/1 -> Product14/2
  Constant5/1 -> Multiply1/1
  Multiply29/1 -> Product29/1
  Multiply51/1 -> Product51/1
  Constant57/1 -> Multiply49/1
  R59/1 -> Product61/2
  Product6/1 -> Simulink-PS Converter10/1
  Multiply90/1 -> Product90/1
  Constant48/1 -> Multiply44/1
  Constant58/1 -> Multiply50/1
  Product8/1 -> Simulink-PS Converter12/1
  R70/1 -> Product72/2
  Multiply81/1 -> Product81/1
  Product59/1 -> Simulink-PS Converter63/1
  Multiply34/1 -> Product34/1
  Multiply42/1 -> Product42/1
  Product43/1 -> Simulink-PS Converter47/1
  R30/1 -> Product29/2
  R21/1 -> Product20/2
  Product49/1 -> Simulink-PS Converter57/1
  Constant19/1 -> Multiply15/1
  Product58/1 -> Simulink-PS Converter62/1
  Constant20/1 -> Multiply16/1
  Product10/1 -> Simulink-PS Converter14/1
  R44/1 -> Product45/2
  R9/1 -> Product8/2
  R57/1 -> Product59/2
  Constant87/1 -> Multiply83/1
  Constant69/1 -> Multiply65/1
  Constant76/1 -> Multiply72/1
  Constant36/1 -> Multiply32/1
  Constant11/1 -> Multiply7/1
  C2/1 -> Product44/2
  R17/1 -> Product16/2
  Constant9/1 -> Multiply5/1
  Product29/1 -> Simulink-PS Converter33/1
  R3/1 -> Product1/2
  Constant89/1 -> Multiply85/1
  Constant45/1 -> Multiply41/1
  R20/1 -> Product19/2
  Product81/1 -> Simulink-PS Converter85/1
  Multiply43/1 -> Product43/1
  Constant29/1 -> Multiply25/1
  Multiply10/1 -> Product10/1
  Product3/1 -> Simulink-PS Converter7/1
  Constant30/1 -> Multiply26/1
  Product33/1 -> Simulink-PS Converter37/1
  Multiply49/1 -> Product49/1
  Multiply33/1 -> Product33/1
  L10/1 -> Product54/2
  Constant37/1 -> Multiply33/1
  Product/1 -> Simulink-PS Converter/1
  Product42/1 -> Simulink-PS Converter46/1
  Constant7/1 -> Multiply3/1
  R34/1 -> Product33/2
  Product41/1 -> Simulink-PS Converter45/1
  Product4/1 -> Simulink-PS Converter8/1
  Constant84/1 -> Multiply80/1
  Product22/1 -> Simulink-PS Converter26/1
  Constant67/1 -> Multiply63/1
  Multiply39/1 -> Product39/1
  R49/1 -> Product50/2
  R62/1 -> Product64/2
  Product63/1 -> Simulink-PS Converter67/1
  R35/1 -> Product34/2
  R2/1 -> Product3/2
  R56/1 -> Product58/2
  Constant46/1 -> Multiply42/1
  Multiply37/1 -> Product37/1
  Constant81/1 -> Multiply77/1
  Multiply3/1 -> Product3/1
  Multiply59/1 -> Product59/1
  Multiply22/1 -> Product22/1
  Multiply36/1 -> Product36/1
  Product91/1 -> Simulink-PS Converter95/1
  Multiply84/1 -> Product84/1
  R4/1 -> Product2/2
  Product87/1 -> Simulink-PS Converter91/1
  Product47/1 -> Simulink-PS Converter55/1
  Product84/1 -> Simulink-PS Converter88/1
  Constant88/1 -> Multiply84/1
  Constant55/1 -> Multiply47/1
  R24/1 -> Product23/2
  Constant16/1 -> Multiply12/1
  Product39/1 -> Simulink-PS Converter43/1
  Multiply35/1 -> Product35/1
  R36/1 -> Product35/2
  R19/1 -> Product18/2
  R14/1 -> Product13/2
  Multiply53/1 -> Product53/1
  Multiply64/1 -> Product64/1
  Constant47/1 -> Multiply43/1
  Product85/1 -> Simulink-PS Converter89/1
  Constant21/1 -> Multiply17/1
  Constant91/1 -> Multiply87/1
  Product38/1 -> Simulink-PS Converter42/1
  R51/1 -> Product52/2
  Constant17/1 -> Multiply13/1
  R11/1 -> Product10/2
  Constant90/1 -> Multiply86/1
  Product28/1 -> Simulink-PS Converter32/1
  Product35/1 -> Simulink-PS Converter39/1
  Product15/1 -> Simulink-PS Converter19/1
  Constant61/1 -> Multiply57/1
  R55/1 -> Product57/2
  R84/1 -> Product86/2
  Multiply52/1 -> Product52/1
  R7/1 -> Product6/2
  Multiply32/1 -> Product32/1
  Constant39/1 -> Multiply35/1
  Product51/1 -> Simulink-PS Converter50/1
  Multiply7/1 -> Product7/1
  Constant38/1 -> Multiply34/1
  Constant6/1 -> Multiply2/1
  Multiply16/1 -> Product16/1
  Product13/1 -> Simulink-PS Converter17/1
  Multiply82/1 -> Product82/1
  Constant65/1 -> Multiply61/1
  Multiply6/1 -> Product6/1
  Multiply62/1 -> Product62/1
  Constant10/1 -> Multiply6/1
  Product55/1 -> Simulink-PS Converter59/1
  R43/1 -> Product42/2
  Constant53/1 -> Multiply54/1
  Constant66/1 -> Multiply62/1
  Multiply1/1 -> Product1/1
  R75/1 -> Product77/2
  Product12/1 -> Simulink-PS Converter16/1
  Multiply26/1 -> Product26/1
  R50/1 -> Product51/2
  Multiply70/1 -> Product70/1
  Product2/1 -> Simulink-PS Converter6/1
  Multiply47/1 -> Product47/1
  Product46/1 -> Simulink-PS Converter54/1
  Product54/1 -> Simulink-PS Converter53/1
  Multiply50/1 -> Product50/1
  Multiply54/1 -> Product54/1
  R29/1 -> Product28/2
  Constant25/1 -> Multiply21/1
  Constant/1 -> Multiply/1
  Product50/1 -> Simulink-PS Converter58/1
  Constant75/1 -> Multiply71/1
  Product16/1 -> Simulink-PS Converter20/1
  R25/1 -> Product24/2
  R52/1 -> Product53/2
  Product77/1 -> Simulink-PS Converter81/1
  Constant52/1 -> Multiply53/1
  Multiply17/1 -> Product17/1
  Multiply68/1 -> Product68/1
  Constant64/1 -> Multiply60/1
  Product86/1 -> Simulink-PS Converter90/1
  Product72/1 -> Simulink-PS Converter76/1
  Product80/1 -> Simulink-PS Converter84/1
  Multiply44/1 -> Product44/1
  Multiply73/1 -> Product73/1
  Multiply65/1 -> Product65/1
  R47/1 -> Product47/2
  Constant73/1 -> Multiply69/1
  Product73/1 -> Simulink-PS Converter77/1
  Constant72/1 -> Multiply68/1
  R28/1 -> Product27/2
  Product69/1 -> Simulink-PS Converter73/1
  Multiply69/1 -> Product69/1
  Product68/1 -> Simulink-PS Converter72/1
  Multiply67/1 -> Product67/1
  R72/1 -> Product74/2
  R5/1 -> Product4/2
  Product67/1 -> Simulink-PS Converter71/1
  Multiply92/1 -> Product92/1
  Constant71/1 -> Multiply67/1
  Abd - L4/1 -> Product91/2
  Constant70/1 -> Multiply66/1
  R37/1 -> Product36/2
  Product66/1 -> Simulink-PS Converter70/1
  Multiply75/1 -> Product75/1
  R69/1 -> Product71/2
  Constant35/1 -> Multiply31/1
  R64/1 -> Product66/2
  Multiply72/1 -> Product72/1
  R71/1 -> Product73/2
  Multiply79/1 -> Product79/1
  Multiply71/1 -> Product71/1
  Constant74/1 -> Multiply70/1
  R65/1 -> Product67/2
  Product14/1 -> Simulink-PS Converter18/1
  Product71/1 -> Simulink-PS Converter75/1
  Multiply78/1 -> Product78/1
  R66/1 -> Product68/2
  Multiply66/1 -> Product66/1
  R68/1 -> Product70/2
  R63/1 -> Product65/2
  Constant59/1 -> Multiply55/1
  R61/1 -> Product63/2
  Constant78/1 -> Multiply74/1
  Product70/1 -> Simulink-PS Converter74/1
  Product74/1 -> Simulink-PS Converter78/1
  Product79/1 -> Simulink-PS Converter83/1
  R85/1 -> Product87/2
  Product21/1 -> Simulink-PS Converter25/1
  Multiply74/1 -> Product74/1
  Constant77/1 -> Multiply73/1
  Product65/1 -> Simulink-PS Converter69/1
  Multiply76/1 -> Product76/1
  Constant86/1 -> Multiply82/1
  Abd - L3/1 -> Product90/2
  Multiply28/1 -> Product28/1
  Product23/1 -> Simulink-PS Converter27/1
  Constant50/1 -> Multiply51/1
  R46/1 -> Product46/2
  Product82/1 -> Simulink-PS Converter86/1
  Multiply48/1 -> Product48/1
  Multiply13/1 -> Product13/1
  Abd - L5/1 -> Product92/2
  Constant54/1 -> Multiply46/1
  Product56/1 -> Simulink-PS Converter60/1
  Multiply46/1 -> Product46/1
  Product45/1 -> Simulink-PS Converter49/1
  Product19/1 -> Simulink-PS Converter23/1
  Product53/1 -> Simulink-PS Converter52/1
  Constant51/1 -> Multiply52/1
  Constant27/1 -> Multiply23/1
  Constant56/1 -> Multiply48/1
  Abd - L2/1 -> Product89/2
  Constant49/1 -> Multiply45/1
  R48/1 -> Product49/2
  R76/1 -> Product78/2
  R45/1 -> Product48/2
  Product11/1 -> Simulink-PS Converter15/1
  Product48/1 -> Simulink-PS Converter56/1
  Constant22/1 -> Multiply18/1
  Constant12/1 -> Multiply8/1
  Constant94/1 -> Multiply90/1
  Multiply8/1 -> Product8/1
  Multiply4/1 -> Product4/1
  Product31/1 -> Simulink-PS Converter35/1
  Product25/1 -> Simulink-PS Converter29/1
  R60/1 -> Product62/2
  R26/1 -> Product25/2
  Multiply38/1 -> Product38/1
  Multiply25/1 -> Product25/1
  R6/1 -> Product5/2
  Multiply41/1 -> Product41/1
  R8/1 -> Product7/2
  Product36/1 -> Simulink-PS Converter40/1
  Constant24/1 -> Multiply20/1
  Product7/1 -> Simulink-PS Converter11/1
  Constant34/1 -> Multiply30/1
  Product18/1 -> Simulink-PS Converter22/1
  Multiply27/1 -> Product27/1
  Product26/1 -> Simulink-PS Converter30/1
  R27/1 -> Product26/2
  R53/1 -> Product55/2
  Product1/1 -> Simulink-PS Converter5/1
  Multiply24/1 -> Product24/1
  Product32/1 -> Simulink-PS Converter36/1
  R33/1 -> Product32/2
  Multiply11/1 -> Product11/1
  R12/1 -> Product11/2
  R18/1 -> Product17/2
  Constant15/1 -> Multiply11/1
  Product44/1 -> Simulink-PS Converter48/1
  R13/1 -> Product12/2
  Constant82/1 -> Multiply78/1
  Product89/1 -> Simulink-PS Converter93/1
  Product9/1 -> Simulink-PS Converter13/1
  Multiply89/1 -> Product89/1
  Multiply12/1 -> Product12/1
  Multiply91/1 -> Product91/1
  R83/1 -> Product85/2
  Constant93/1 -> Multiply89/1
  Product37/1 -> Simulink-PS Converter41/1
  R22/1 -> Product21/2
  R38/1 -> Product37/2
  R42/1 -> Product41/2
  Multiply21/1 -> Product21/1
  R58/1 -> Product60/2
  Product64/1 -> Simulink-PS Converter68/1
  R82/1 -> Product84/2
  Constant14/1 -> Multiply10/1
  Product20/1 -> Simulink-PS Converter24/1
  Multiply60/1 -> Product60/1
  Multiply20/1 -> Product20/1
  Product57/1 -> Simulink-PS Converter61/1
  R39/1 -> Product38/2
  Multiply40/1 -> Product40/1
  Constant42/1 -> Multiply38/1
  Multiply31/1 -> Product31/1
  Product5/1 -> Simulink-PS Converter9/1
  Multiply86/1 -> Product86/1
  Multiply5/1 -> Product5/1
  Constant68/1 -> Multiply64/1
  Constant96/1 -> Multiply92/1
  Product27/1 -> Simulink-PS Converter31/1
  Product61/1 -> Simulink-PS Converter65/1
  Multiply63/1 -> Product63/1
  R1/1 -> Product/2
  R81/1 -> Product83/2
  R32/1 -> Product31/2
  Multiply/1 -> Product/1
  Product62/1 -> Simulink-PS Converter66/1
  Multiply61/1 -> Product61/1
  Constant63/1 -> Multiply59/1
  Product60/1 -> Simulink-PS Converter64/1
  R23/1 -> Product22/2
  Multiply77/1 -> Product77/1
  Constant60/1 -> Multiply56/1
  Multiply55/1 -> Product55/1
  R54/1 -> Product56/2
  Multiply57/1 -> Product57/1
  Constant62/1 -> Multiply58/1
  Multiply56/1 -> Product56/1
  Multiply58/1 -> Product58/1
  R79/1 -> Product81/2
  Constant26/1 -> Multiply22/1
  Multiply88/1 -> Product88/1
  Multiply19/1 -> Product19/1
  Product90/1 -> Simulink-PS Converter94/1
  Constant23/1 -> Multiply19/1
  Constant28/1 -> Multiply24/1
  Product24/1 -> Simulink-PS Converter28/1
  Multiply83/1 -> Product83/1
  R10/1 -> Product9/2
  Multiply2/1 -> Product2/1
  R74/1 -> Product76/2
  Constant18/1 -> Multiply14/1
  Multiply87/1 -> Product87/1
  Product40/1 -> Simulink-PS Converter44/1
  R41/1 -> Product40/2
  Constant44/1 -> Multiply40/1
  Constant41/1 -> Multiply37/1
  Constant40/1 -> Multiply36/1
  Constant32/1 -> Multiply28/1
  Multiply18/1 -> Product18/1
  Multiply85/1 -> Product85/1
  R73/1 -> Product75/2
  Product83/1 -> Simulink-PS Converter87/1
  Constant31/1 -> Multiply27/1
  Constant80/1 -> Multiply76/1
  R80/1 -> Product82/2
  Product76/1 -> Simulink-PS Converter80/1
  R77/1 -> Product79/2
  Constant83/1 -> Multiply79/1
  Multiply80/1 -> Product80/1
  Product78/1 -> Simulink-PS Converter82/1
  Product92/1 -> Simulink-PS Converter96/1
  Constant79/1 -> Multiply75/1
  Product75/1 -> Simulink-PS Converter79/1
  Multiply15/1 -> Product15/1
  R16/1 -> Product15/2
  Multiply9/1 -> Product9/1
  Constant13/1 -> Multiply9/1
  Constant43/1 -> Multiply39/1
  R40/1 -> Product39/2
  Abd - L1/1 -> Product88/2
  Product88/1 -> Simulink-PS Converter92/1
  Constant92/1 -> Multiply88/1
  Product30/1 -> Simulink-PS Converter34/1
  R31/1 -> Product30/2
  Multiply30/1 -> Product30/1
  Constant1/1 -> Product90/3, Product91/3, Product92/3, Product88/3, Product89/3
  connections:
  External Force and Torque78/RConn1 -- File Solid2/RConn35
  External Force and Torque40/RConn1 -- File Solid2/LConn42
  External Force and Torque18/RConn1 -- File Solid2/LConn20
  External Force and Torque32/RConn1 -- File Solid2/LConn34
  Simulink-PS Converter72/RConn1 -- External Force and Torque68/LConn1
  External Force and Torque27/RConn1 -- File Solid2/LConn29
  External Force and Torque67/RConn1 -- File Solid2/RConn24
  External Force and Torque44/RConn1 -- File Solid2/RConn45
  File Solid2/LConn1 -- To L1/RConn1
  Simulink-PS Converter37/RConn1 -- External Force and Torque33/LConn1
  External Force and Torque39/RConn1 -- File Solid2/LConn41
  External Force and Torque57/RConn1 -- File Solid2/RConn14
  Simulink-PS Converter33/RConn1 -- External Force and Torque29/LConn1
  Simulink-PS Converter43/RConn1 -- External Force and Torque39/LConn1
  Simulink-PS Converter/RConn1 -- External Force and Torque/LConn1
  External Force and Torque58/RConn1 -- File Solid2/RConn15
  External Force and Torque1/RConn1 -- File Solid2/LConn4
  External Force and Torque11/RConn1 -- File Solid2/LConn13
  External Force and Torque63/RConn1 -- File Solid2/RConn20
  External Force and Torque14/RConn1 -- File Solid2/LConn16
  External Force and Torque65/RConn1 -- File Solid2/RConn22
  Simulink-PS Converter96/RConn1 -- External Force and Torque92/LConn1
  Simulink-PS Converter90/RConn1 -- External Force and Torque86/LConn1
  Simulink-PS Converter67/RConn1 -- External Force and Torque63/LConn1
  External Force and Torque75/RConn1 -- File Solid2/RConn32
  Simulink-PS Converter77/RConn1 -- External Force and Torque73/LConn1
  Simulink-PS Converter56/RConn1 -- External Force and Torque48/LConn1
  Simulink-PS Converter10/RConn1 -- External Force and Torque6/LConn1
  Simulink-PS Converter9/RConn1 -- External Force and Torque5/LConn1
  Simulink-PS Converter21/RConn1 -- External Force and Torque17/LConn1
  Simulink-PS Converter64/RConn1 -- External Force and Torque60/LConn1
  Simulink-PS Converter75/RConn1 -- External Force and Torque71/LConn1
  External Force and Torque52/RConn1 -- File Solid2/RConn9
  Simulink-PS Converter39/RConn1 -- External Force and Torque35/LConn1
  Simulink-PS Converter7/RConn1 -- External Force and Torque3/LConn1
  Simulink-PS Converter93/RConn1 -- External Force and Torque89/LConn1
  External Force and Torque5/RConn1 -- File Solid2/LConn7
  External Force and Torque20/RConn1 -- File Solid2/LConn22
  External Force and Torque79/RConn1 -- File Solid2/RConn36
  External Force and Torque35/RConn1 -- File Solid2/LConn37
  External Force and Torque3/RConn1 -- File Solid2/LConn3
  External Force and Torque38/RConn1 -- File Solid2/LConn40
  Simulink-PS Converter26/RConn1 -- External Force and Torque22/LConn1
  External Force and Torque91/RConn1 -- To L2 CONE/RConn1
  Simulink-PS Converter47/RConn1 -- External Force and Torque43/LConn1
  Simulink-PS Converter94/RConn1 -- External Force and Torque90/LConn1
  External Force and Torque61/RConn1 -- File Solid2/RConn18
  External Force and Torque4/RConn1 -- File Solid2/LConn6
  External Force and Torque92/RConn1 -- To L1 CONE/RConn1
  Simulink-PS Converter54/RConn1 -- External Force and Torque46/LConn1
  External Force and Torque62/RConn1 -- File Solid2/RConn19
  External Force and Torque45/RConn1 -- File Solid2/RConn2
  External Force and Torque59/RConn1 -- File Solid2/RConn16
  Simulink-PS Converter91/RConn1 -- External Force and Torque87/LConn1
  External Force and Torque84/RConn1 -- File Solid2/RConn41
  Simulink-PS Converter62/RConn1 -- External Force and Torque58/LConn1
  Simulink-PS Converter50/RConn1 -- External Force and Torque51/LConn1
  Simulink-PS Converter38/RConn1 -- External Force and Torque34/LConn1
  Simulink-PS Converter83/RConn1 -- External Force and Torque79/LConn1
  Simulink-PS Converter52/RConn1 -- External Force and Torque53/LConn1
  Simulink-PS Converter74/RConn1 -- External Force and Torque70/LConn1
  External Force and Torque24/RConn1 -- File Solid2/LConn26
  External Force and Torque66/RConn1 -- File Solid2/RConn23
  External Force and Torque55/RConn1 -- File Solid2/RConn12
  External Force and Torque42/RConn1 -- File Solid2/LConn44
  Simulink-PS Converter70/RConn1 -- External Force and Torque66/LConn1
  Simulink-PS Converter51/RConn1 -- External Force and Torque52/LConn1
  Simulink-PS Converter46/RConn1 -- External Force and Torque42/LConn1
  Simulink-PS Converter66/RConn1 -- External Force and Torque62/LConn1
  Simulink-PS Converter49/RConn1 -- External Force and Torque45/LConn1
  External Force and Torque31/RConn1 -- File Solid2/LConn33
  Simulink-PS Converter71/RConn1 -- External Force and Torque67/LConn1
  Simulink-PS Converter57/RConn1 -- External Force and Torque49/LConn1
  External Force and Torque12/RConn1 -- File Solid2/LConn14
  Simulink-PS Converter20/RConn1 -- External Force and Torque16/LConn1
  Simulink-PS Converter55/RConn1 -- External Force and Torque47/LConn1
  Simulink-PS Converter58/RConn1 -- External Force and Torque50/LConn1
  External Force and Torque77/RConn1 -- File Solid2/RConn34
  Simulink-PS Converter53/RConn1 -- External Force and Torque54/LConn1
  External Force and Torque17/RConn1 -- File Solid2/LConn19
  External Force and Torque2/RConn1 -- File Solid2/LConn5
  Simulink-PS Converter76/RConn1 -- External Force and Torque72/LConn1
  External Force and Torque51/RConn1 -- File Solid2/RConn8
  Simulink-PS Converter23/RConn1 -- External Force and Torque19/LConn1
  Simulink-PS Converter69/RConn1 -- External Force and Torque65/LConn1
  Simulink-PS Converter78/RConn1 -- External Force and Torque74/LConn1
  Simulink-PS Converter73/RConn1 -- External Force and Torque69/LConn1
  External Force and Torque74/RConn1 -- File Solid2/RConn31
  External Force and Torque8/RConn1 -- File Solid2/LConn10
  Simulink-PS Converter12/RConn1 -- External Force and Torque8/LConn1
  Simulink-PS Converter28/RConn1 -- External Force and Torque24/LConn1
  Simulink-PS Converter45/RConn1 -- External Force and Torque41/LConn1
  External Force and Torque54/RConn1 -- File Solid2/RConn11
  Simulink-PS Converter11/RConn1 -- External Force and Torque7/LConn1
  Simulink-PS Converter59/RConn1 -- External Force and Torque55/LConn1
  External Force and Torque6/RConn1 -- File Solid2/LConn8
  Simulink-PS Converter5/RConn1 -- External Force and Torque1/LConn1
  External Force and Torque7/RConn1 -- File Solid2/LConn9
  External Force and Torque60/RConn1 -- File Solid2/RConn17
  External Force and Torque10/RConn1 -- File Solid2/LConn12
  Simulink-PS Converter24/RConn1 -- External Force and Torque20/LConn1
  External Force and Torque53/RConn1 -- File Solid2/RConn10
  External Force and Torque21/RConn1 -- File Solid2/LConn23
  External Force and Torque89/RConn1 -- To L4 CONE/RConn1
  External Force and Torque43/RConn1 -- File Solid2/LConn45
  External Force and Torque72/RConn1 -- File Solid2/RConn29
  External Force and Torque48/RConn1 -- File Solid2/RConn3
  External Force and Torque47/RConn1 -- File Solid2/RConn5
  External Force and Torque70/RConn1 -- File Solid2/RConn27
  External Force and Torque69/RConn1 -- File Solid2/RConn26
  External Force and Torque22/RConn1 -- File Solid2/LConn24
  External Force and Torque49/RConn1 -- File Solid2/RConn6
  External Force and Torque37/RConn1 -- File Solid2/LConn39
  External Force and Torque46/RConn1 -- File Solid2/RConn4
  External Force and Torque50/RConn1 -- File Solid2/RConn7
  External Force and Torque30/RConn1 -- File Solid2/LConn32
  Simulink-PS Converter17/RConn1 -- External Force and Torque13/LConn1
  External Force and Torque26/RConn1 -- File Solid2/LConn28
  External Force and Torque9/RConn1 -- File Solid2/LConn11
  Simulink-PS Converter95/RConn1 -- External Force and Torque91/LConn1
  Simulink-PS Converter29/RConn1 -- External Force and Torque25/LConn1
  External Force and Torque82/RConn1 -- File Solid2/RConn39
  External Force and Torque80/RConn1 -- File Solid2/RConn37
  Simulink-PS Converter40/RConn1 -- External Force and Torque36/LConn1
  External Force and Torque29/RConn1 -- File Solid2/LConn31
  Simulink-PS Converter27/RConn1 -- External Force and Torque23/LConn1
  External Force and Torque71/RConn1 -- File Solid2/RConn28
  External Force and Torque68/RConn1 -- File Solid2/RConn25
  Simulink-PS Converter65/RConn1 -- External Force and Torque61/LConn1
  Simulink-PS Converter30/RConn1 -- External Force and Torque26/LConn1
  External Force and Torque16/RConn1 -- File Solid2/LConn18
  External Force and Torque81/RConn1 -- File Solid2/RConn38
  External Force and Torque28/RConn1 -- File Solid2/LConn30
  Simulink-PS Converter36/RConn1 -- External Force and Torque32/LConn1
  Simulink-PS Converter48/RConn1 -- External Force and Torque44/LConn1
  Simulink-PS Converter15/RConn1 -- External Force and Torque11/LConn1
  Simulink-PS Converter88/RConn1 -- External Force and Torque84/LConn1
  External Force and Torque64/RConn1 -- File Solid2/RConn21
  External Force and Torque86/RConn1 -- File Solid2/RConn43
  Simulink-PS Converter32/RConn1 -- External Force and Torque28/LConn1
  Simulink-PS Converter14/RConn1 -- External Force and Torque10/LConn1
  Simulink-PS Converter25/RConn1 -- External Force and Torque21/LConn1
  External Force and Torque76/RConn1 -- File Solid2/RConn33
  Simulink-PS Converter42/RConn1 -- External Force and Torque38/LConn1
  Simulink-PS Converter61/RConn1 -- External Force and Torque57/LConn1
  External Force and Torque83/RConn1 -- File Solid2/RConn40
  Simulink-PS Converter35/RConn1 -- External Force and Torque31/LConn1
  External Force and Torque/RConn1 -- File Solid2/LConn2
  Simulink-PS Converter60/RConn1 -- External Force and Torque56/LConn1
  Simulink-PS Converter63/RConn1 -- External Force and Torque59/LConn1
  Simulink-PS Converter68/RConn1 -- External Force and Torque64/LConn1
  External Force and Torque85/RConn1 -- File Solid2/RConn42
  Simulink-PS Converter34/RConn1 -- External Force and Torque30/LConn1
  Simulink-PS Converter8/RConn1 -- External Force and Torque4/LConn1
  External Force and Torque90/RConn1 -- To L3 CONE/RConn1
  Simulink-PS Converter16/RConn1 -- External Force and Torque12/LConn1
  External Force and Torque34/RConn1 -- File Solid2/LConn36
  External Force and Torque87/RConn1 -- File Solid2/RConn44
  External Force and Torque23/RConn1 -- File Solid2/LConn25
  External Force and Torque36/RConn1 -- File Solid2/LConn38
  Simulink-PS Converter6/RConn1 -- External Force and Torque2/LConn1
  Simulink-PS Converter44/RConn1 -- External Force and Torque40/LConn1
  External Force and Torque19/RConn1 -- File Solid2/LConn21
  Simulink-PS Converter18/RConn1 -- External Force and Torque14/LConn1
  External Force and Torque25/RConn1 -- File Solid2/LConn27
  Simulink-PS Converter41/RConn1 -- External Force and Torque37/LConn1
  External Force and Torque41/RConn1 -- File Solid2/LConn43
  External Force and Torque13/RConn1 -- File Solid2/LConn15
  Simulink-PS Converter22/RConn1 -- External Force and Torque18/LConn1
  Simulink-PS Converter89/RConn1 -- External Force and Torque85/LConn1
  Simulink-PS Converter87/RConn1 -- External Force and Torque83/LConn1
  Simulink-PS Converter79/RConn1 -- External Force and Torque75/LConn1
  Simulink-PS Converter31/RConn1 -- External Force and Torque27/LConn1
  Simulink-PS Converter85/RConn1 -- External Force and Torque81/LConn1
  Simulink-PS Converter81/RConn1 -- External Force and Torque77/LConn1
  External Force and Torque73/RConn1 -- File Solid2/RConn30
  Simulink-PS Converter86/RConn1 -- External Force and Torque82/LConn1
  Simulink-PS Converter80/RConn1 -- External Force and Torque76/LConn1
  Simulink-PS Converter84/RConn1 -- External Force and Torque80/LConn1
  Simulink-PS Converter82/RConn1 -- External Force and Torque78/LConn1
  Simulink-PS Converter19/RConn1 -- External Force and Torque15/LConn1
  External Force and Torque33/RConn1 -- File Solid2/LConn35
  Simulink-PS Converter13/RConn1 -- External Force and Torque9/LConn1
  Simulink-PS Converter92/RConn1 -- External Force and Torque88/LConn1
  External Force and Torque56/RConn1 -- File Solid2/RConn13
  External Force and Torque15/RConn1 -- File Solid2/LConn17
  External Force and Torque88/RConn1 -- To L5 CONE/RConn1
